simulink model "ARINC429_BNR"  (R2020b)
settings: Solver=VariableStepAuto  StartTime=0.0  StopTime=10.0  RelTol=1e-3
libraries: Bibavion x1
(part 2 of 3)

== system ARINC429_BNR/Decoder/De-serialize/Subsystem29 ==
  In1 : Inport
  Data Type Conversion5 : DataTypeConversion  OutDataTypeStr=uint32
  Data Type Conversion9 : DataTypeConversion  OutDataTypeStr=uint32
  Divide12 : Product  Inputs=*/
  Divide13 : Product  Inputs=*/  OutDataTypeStr=uint32
  Float Const : Constant  Value=2  OutDataTypeStr=single
  Float Const6 : Constant  Value=0.5  OutDataTypeStr=single
  Subtract5 : Sum  Inputs=+-
  Out1 : Outport
  Out2 : Outport  Port=2
  wires:
  Float Const/1 -> [F_2]
  Divide12/1 -> Subtract5/1, Data Type Conversion5/1
  Divide13/1 -> Data Type Conversion9/1
  Float Const6/1 -> Divide13/2
  Data Type Conversion5/1 -> Out2/1, Subtract5/2
  [F_2] -> Divide12/2
  Subtract5/1 -> Divide13/1
  Data Type Conversion9/1 -> Out1/1
  In1/1 -> Divide12/1

== system ARINC429_BNR/Decoder/De-serialize/Subsystem3 ==
  In1 : Inport
  Data Type Conversion5 : DataTypeConversion  OutDataTypeStr=uint32
  Data Type Conversion9 : DataTypeConversion  OutDataTypeStr=uint32
  Divide12 : Product  Inputs=*/  OutDataTypeStr=double
  Divide13 : Product  Inputs=*/
  Float Const : Constant  Value=2  OutDataTypeStr=single
  Float Const6 : Constant  Value=0.5  OutDataTypeStr=single
  Subtract5 : Sum  Inputs=+-
  Out1 : Outport
  Out2 : Outport  Port=2
  wires:
  Float Const/1 -> [F_2]
  Divide12/1 -> Subtract5/1, Data Type Conversion5/1
  Divide13/1 -> Data Type Conversion9/1
  Float Const6/1 -> Divide13/2
  Data Type Conversion5/1 -> Out2/1, Subtract5/2
  In1/1 -> Divide12/1
  [F_2] -> Divide12/2
  Subtract5/1 -> Divide13/1
  Data Type Conversion9/1 -> Out1/1

== system ARINC429_BNR/Decoder/De-serialize/Subsystem30 ==
  In1 : Inport
  Data Type Conversion5 : DataTypeConversion  OutDataTypeStr=uint32
  Data Type Conversion9 : DataTypeConversion  OutDataTypeStr=uint32
  Divide12 : Product  Inputs=*/
  Divide13 : Product  Inputs=*/  OutDataTypeStr=uint32
  Float Const : Constant  Value=2  OutDataTypeStr=single
  Float Const6 : Constant  Value=0.5  OutDataTypeStr=single
  Subtract5 : Sum  Inputs=+-
  Out1 : Outport
  Out2 : Outport  Port=2
  wires:
  Float Const/1 -> [F_2]
  Divide12/1 -> Subtract5/1, Data Type Conversion5/1
  Divide13/1 -> Data Type Conversion9/1
  Float Const6/1 -> Divide13/2
  Data Type Conversion5/1 -> Out2/1, Subtract5/2
  [F_2] -> Divide12/2
  Subtract5/1 -> Divide13/1
  Data Type Conversion9/1 -> Out1/1
  In1/1 -> Divide12/1

== system ARINC429_BNR/Decoder/De-serialize/Subsystem31 ==
  In1 : Inport
  Data Type Conversion5 : DataTypeConversion  OutDataTypeStr=uint32
  Data Type Conversion9 : DataTypeConversion  OutDataTypeStr=uint32
  Divide12 : Product  Inputs=*/
  Divide13 : Product  Inputs=*/  OutDataTypeStr=uint32
  Float Const : Constant  Value=2  OutDataTypeStr=single
  Float Const6 : Constant  Value=0.5  OutDataTypeStr=single
  Subtract5 : Sum  Inputs=+-
  Out1 : Outport
  Out2 : Outport  Port=2
  wires:
  Float Const/1 -> [F_2]
  Divide12/1 -> Subtract5/1, Data Type Conversion5/1
  Divide13/1 -> Data Type Conversion9/1
  Float Const6/1 -> Divide13/2
  Data Type Conversion5/1 -> Out2/1, Subtract5/2
  [F_2] -> Divide12/2
  Subtract5/1 -> Divide13/1
  Data Type Conversion9/1 -> Out1/1
  In1/1 -> Divide12/1

== system ARINC429_BNR/Decoder/De-serialize/Subsystem32 ==
  In1 : Inport
  Data Type Conversion5 : DataTypeConversion  OutDataTypeStr=uint32
  Data Type Conversion9 : DataTypeConversion  OutDataTypeStr=uint32
  Divide12 : Product  Inputs=*/
  Divide13 : Product  Inputs=*/  OutDataTypeStr=uint32
  Float Const : Constant  Value=2  OutDataTypeStr=single
  Float Const6 : Constant  Value=0.5  OutDataTypeStr=single
  Subtract5 : Sum  Inputs=+-
  Out1 : Outport
  Out2 : Outport  Port=2
  wires:
  Float Const/1 -> [F_2]
  Divide12/1 -> Subtract5/1, Data Type Conversion5/1
  Divide13/1 -> Data Type Conversion9/1
  Float Const6/1 -> Divide13/2
  Data Type Conversion5/1 -> Out2/1, Subtract5/2
  [F_2] -> Divide12/2
  Subtract5/1 -> Divide13/1
  Data Type Conversion9/1 -> Out1/1
  In1/1 -> Divide12/1

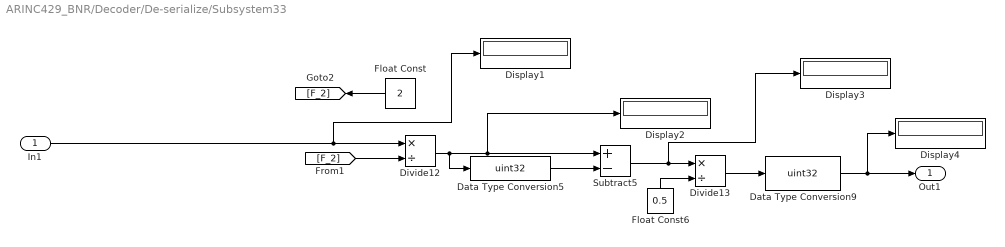
== system ARINC429_BNR/Decoder/De-serialize/Subsystem33 ==
  In1 : Inport
  Data Type Conversion5 : DataTypeConversion  OutDataTypeStr=uint32
  Data Type Conversion9 : DataTypeConversion  OutDataTypeStr=uint32
  Display{1..4} (4 alike) : Display
      settings: Format=decimal (Stored Integer)
  Divide12 : Product  Inputs=*/  OutDataTypeStr=double
  Divide13 : Product  Inputs=*/  OutDataTypeStr=uint32
  Float Const : Constant  Value=2  OutDataTypeStr=single
  Float Const6 : Constant  Value=0.5  OutDataTypeStr=single
  Subtract5 : Sum  Inputs=+-
  Out1 : Outport
  wires:
  Float Const/1 -> [F_2]
  Divide12/1 -> Display2/1, Subtract5/1, Data Type Conversion5/1
  Divide13/1 -> Data Type Conversion9/1
  Float Const6/1 -> Divide13/2
  Data Type Conversion5/1 -> Subtract5/2
  [F_2] -> Divide12/2
  Subtract5/1 -> Display3/1, Divide13/1
  Data Type Conversion9/1 -> Display4/1, Out1/1
  In1/1 -> Display1/1, Divide12/1

== system ARINC429_BNR/Decoder/De-serialize/Subsystem4 ==
  In1 : Inport
  Data Type Conversion5 : DataTypeConversion  OutDataTypeStr=uint32
  Data Type Conversion9 : DataTypeConversion  OutDataTypeStr=uint32
  Divide12 : Product  Inputs=*/  OutDataTypeStr=double
  Divide13 : Product  Inputs=*/  OutDataTypeStr=uint32
  Float Const : Constant  Value=2  OutDataTypeStr=single
  Float Const6 : Constant  Value=0.5  OutDataTypeStr=single
  Subtract5 : Sum  Inputs=+-
  Out1 : Outport
  Out2 : Outport  Port=2
  wires:
  Float Const/1 -> [F_2]
  Divide12/1 -> Subtract5/1, Data Type Conversion5/1
  Divide13/1 -> Data Type Conversion9/1
  Float Const6/1 -> Divide13/2
  Data Type Conversion5/1 -> Out2/1, Subtract5/2
  [F_2] -> Divide12/2
  Subtract5/1 -> Divide13/1
  Data Type Conversion9/1 -> Out1/1
  In1/1 -> Divide12/1

== system ARINC429_BNR/Decoder/De-serialize/Subsystem7 ==
  In1 : Inport
  Data Type Conversion5 : DataTypeConversion  OutDataTypeStr=uint32
  Data Type Conversion9 : DataTypeConversion  OutDataTypeStr=uint32
  Divide12 : Product  Inputs=*/  OutDataTypeStr=double
  Divide13 : Product  Inputs=*/  OutDataTypeStr=uint32
  Float Const : Constant  Value=2  OutDataTypeStr=single
  Float Const6 : Constant  Value=0.5  OutDataTypeStr=single
  Subtract5 : Sum  Inputs=+-
  Out1 : Outport
  Out2 : Outport  Port=2
  wires:
  Float Const/1 -> [F_2]
  Divide12/1 -> Subtract5/1, Data Type Conversion5/1
  Divide13/1 -> Data Type Conversion9/1
  Float Const6/1 -> Divide13/2
  Data Type Conversion5/1 -> Out2/1, Subtract5/2
  [F_2] -> Divide12/2
  Subtract5/1 -> Divide13/1
  Data Type Conversion9/1 -> Out1/1
  In1/1 -> Divide12/1

== system ARINC429_BNR/Decoder/De-serialize/Subsystem8 ==
  In1 : Inport
  Data Type Conversion5 : DataTypeConversion  OutDataTypeStr=uint32
  Data Type Conversion9 : DataTypeConversion  OutDataTypeStr=uint32
  Divide12 : Product  Inputs=*/  OutDataTypeStr=double
  Divide13 : Product  Inputs=*/  OutDataTypeStr=uint32
  Float Const : Constant  Value=2  OutDataTypeStr=single
  Float Const6 : Constant  Value=0.5  OutDataTypeStr=single
  Subtract5 : Sum  Inputs=+-
  Out1 : Outport
  Out2 : Outport  Port=2
  wires:
  Float Const/1 -> [F_2]
  Divide12/1 -> Subtract5/1, Data Type Conversion5/1
  Divide13/1 -> Data Type Conversion9/1
  Float Const6/1 -> Divide13/2
  Data Type Conversion5/1 -> Out2/1, Subtract5/2
  [F_2] -> Divide12/2
  Subtract5/1 -> Divide13/1
  Data Type Conversion9/1 -> Out1/1
  In1/1 -> Divide12/1

== system ARINC429_BNR/Decoder/De-serialize/Subsystem9 ==
  In1 : Inport
  Data Type Conversion5 : DataTypeConversion  OutDataTypeStr=uint32
  Data Type Conversion9 : DataTypeConversion  OutDataTypeStr=uint32
  Divide12 : Product  Inputs=*/  OutDataTypeStr=double
  Divide13 : Product  Inputs=*/  OutDataTypeStr=uint32
  Float Const : Constant  Value=2  OutDataTypeStr=single
  Float Const6 : Constant  Value=0.5  OutDataTypeStr=single
  Subtract5 : Sum  Inputs=+-
  Out1 : Outport
  Out2 : Outport  Port=2
  wires:
  Float Const/1 -> [F_2]
  Divide12/1 -> Subtract5/1, Data Type Conversion5/1
  Divide13/1 -> Data Type Conversion9/1
  Float Const6/1 -> Divide13/2
  Data Type Conversion5/1 -> Out2/1, Subtract5/2
  [F_2] -> Divide12/2
  Subtract5/1 -> Divide13/1
  Data Type Conversion9/1 -> Out1/1
  In1/1 -> Divide12/1

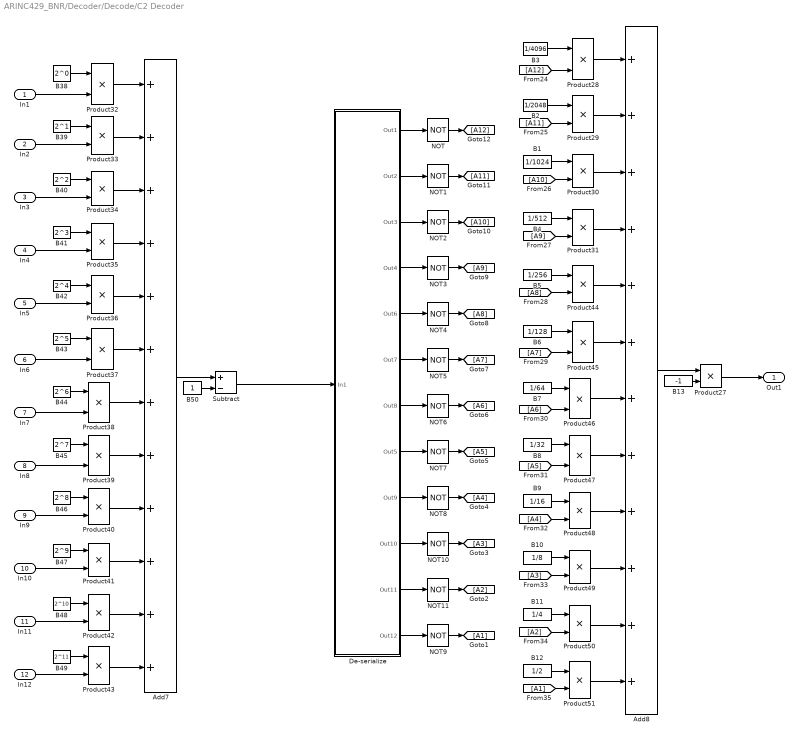
== system ARINC429_BNR/Decoder/Decode/C2 Decoder ==
  In1 : Inport
  In2 : Inport  Port=2
  In3 : Inport  Port=3
  In4 : Inport  Port=4
  In5 : Inport  Port=5
  In6 : Inport  Port=6
  In7 : Inport  Port=7
  In8 : Inport  Port=8
  In9 : Inport  Port=9
  In10 : Inport  Port=10
  In11 : Inport  Port=11
  In12 : Inport  Port=12
  Add7 : Sum  Inputs=++++++++++++  AccumDataTypeStr=uint32  OutDataTypeStr=uint32
  Add8 : Sum  Inputs=++++++++++++
  B1 : Constant  Value=1/1024  OutDataTypeStr=single
  B10 : Constant  Value=1/8  OutDataTypeStr=single
  B11 : Constant  Value=1/4  OutDataTypeStr=single
  B12 : Constant  Value=1/2  OutDataTypeStr=single
  B13 : Constant  Value=-1  OutDataTypeStr=single
  B2 : Constant  Value=1/2048  OutDataTypeStr=single
  B3 : Constant  Value=1/4096  OutDataTypeStr=single
  B38 : Constant  Value=2^0  OutDataTypeStr=single
  B39 : Constant  Value=2^1  OutDataTypeStr=single
  B4 : Constant  Value=1/512  OutDataTypeStr=single
  B40 : Constant  Value=2^2  OutDataTypeStr=single
  B41 : Constant  Value=2^3  OutDataTypeStr=single
  B42 : Constant  Value=2^4  OutDataTypeStr=single
  B43 : Constant  Value=2^5  OutDataTypeStr=single
  B44 : Constant  Value=2^6  OutDataTypeStr=single
  B45 : Constant  Value=2^7  OutDataTypeStr=single
  B46 : Constant  Value=2^8  OutDataTypeStr=single
  B47 : Constant  Value=2^9  OutDataTypeStr=single
  B48 : Constant  Value=2^10  OutDataTypeStr=single
  B49 : Constant  Value=2^11  OutDataTypeStr=single
  B5 : Constant  Value=1/256  OutDataTypeStr=single
  B50 : Constant  OutDataTypeStr=single
  B6 : Constant  Value=1/128  OutDataTypeStr=single
  B7 : Constant  Value=1/64  OutDataTypeStr=single
  B8 : Constant  Value=1/32  OutDataTypeStr=single
  B9 : Constant  Value=1/16  OutDataTypeStr=single
  De-serialize : Subsystem
  NOT{,1..11} (12 alike) : Logic  Operator=NOT  IconShape=distinctive  AllPortsSameDT=off  OutDataTypeStr=boolean
  Product{27..51} (25 alike) : Product
  Subtract : Sum  Inputs=+-
  Out1 : Outport
  wires:
  B41/1 -> Product35/1
  NOT1/1 -> [A11]
  De-serialize/12(Out12) -> NOT9/1
  [A12] -> Product28/2
  De-serialize/7(Out8) -> NOT6/1
  B48/1 -> Product42/1
  [A7] -> Product45/2
  Product30/1 -> Add8/3
  B44/1 -> Product38/1
  B42/1 -> Product36/1
  B49/1 -> Product43/1
  Product31/1 -> Add8/4
  Product42/1 -> Add7/11
  De-serialize/8(Out5) -> NOT7/1
  B46/1 -> Product40/1
  [A5] -> Product47/2
  NOT10/1 -> [A3]
  Product36/1 -> Add7/5
  B3/1 -> Product28/1
  NOT/1 -> [A12]
  Product41/1 -> Add7/10
  De-serialize/6(Out7) -> NOT5/1
  B45/1 -> Product39/1
  De-serialize/1(Out1) -> NOT/1
  NOT3/1 -> [A9]
  [A6] -> Product46/2
  Product44/1 -> Add8/5
  De-serialize/11(Out11) -> NOT11/1
  [A10] -> Product30/2
  Product35/1 -> Add7/4
  Product51/1 -> Add8/12
  Product43/1 -> Add7/12
  Product47/1 -> Add8/8
  In12/1 -> Product43/2
  NOT8/1 -> [A4]
  B11/1 -> Product50/1
  Subtract/1 -> De-serialize/1(In1)
  NOT2/1 -> [A10]
  [A1] -> Product51/2
  B38/1 -> Product32/1
  [A3] -> Product49/2
  B47/1 -> Product41/1
  De-serialize/4(Out4) -> NOT3/1
  Product37/1 -> Add7/6
  B1/1 -> Product30/1
  B9/1 -> Product48/1
  Product32/1 -> Add7/1
  Product34/1 -> Add7/3
  B39/1 -> Product33/1
  De-serialize/2(Out2) -> NOT1/1
  NOT9/1 -> [A1]
  De-serialize/3(Out3) -> NOT2/1
  [A9] -> Product31/2
  Product39/1 -> Add7/8
  Add7/1 -> Subtract/1
  [A11] -> Product29/2
  NOT11/1 -> [A2]
  B10/1 -> Product49/1
  B40/1 -> Product34/1
  B4/1 -> Product31/1
  Product33/1 -> Add7/2
  B50/1 -> Subtract/2
  NOT7/1 -> [A5]
  De-serialize/9(Out9) -> NOT8/1
  De-serialize/5(Out6) -> NOT4/1
  Product38/1 -> Add7/7
  B43/1 -> Product37/1
  Product40/1 -> Add7/9
  NOT5/1 -> [A7]
  B5/1 -> Product44/1
  B7/1 -> Product46/1
  Product48/1 -> Add8/9
  NOT4/1 -> [A8]
  De-serialize/10(Out10) -> NOT10/1
  B6/1 -> Product45/1
  Product46/1 -> Add8/7
  In2/1 -> Product33/2
  Product50/1 -> Add8/11
  Product45/1 -> Add8/6
  Product28/1 -> Add8/1
  Product29/1 -> Add8/2
  B8/1 -> Product47/1
  B12/1 -> Product51/1
  Product49/1 -> Add8/10
  [A2] -> Product50/2
  [A4] -> Product48/2
  B2/1 -> Product29/1
  [A8] -> Product44/2
  NOT6/1 -> [A6]
  In8/1 -> Product39/2
  In9/1 -> Product40/2
  In5/1 -> Product36/2
  In3/1 -> Product34/2
  In7/1 -> Product38/2
  In4/1 -> Product35/2
  In1/1 -> Product32/2
  In6/1 -> Product37/2
  In11/1 -> Product42/2
  In10/1 -> Product41/2
  Add8/1 -> Product27/1
  Product27/1 -> Out1/1
  B13/1 -> Product27/2

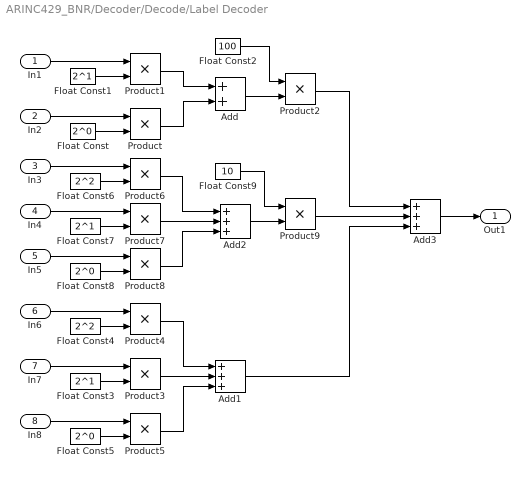
== system ARINC429_BNR/Decoder/Decode/Label Decoder ==
  In1 : Inport
  In2 : Inport  Port=2
  In3 : Inport  Port=3
  In4 : Inport  Port=4
  In5 : Inport  Port=5
  In6 : Inport  Port=6
  In7 : Inport  Port=7
  In8 : Inport  Port=8
  Add : Sum
  Add1 : Sum  Inputs=+++
  Add2 : Sum  Inputs=+++
  Add3 : Sum  Inputs=+++
  Float Const : Constant  Value=2^0  OutDataTypeStr=single
  Float Const1 : Constant  Value=2^1  OutDataTypeStr=single
  Float Const2 : Constant  Value=100  OutDataTypeStr=single
  Float Const3 : Constant  Value=2^1  OutDataTypeStr=single
  Float Const4 : Constant  Value=2^2  OutDataTypeStr=single
  Float Const5 : Constant  Value=2^0  OutDataTypeStr=single
  Float Const6 : Constant  Value=2^2  OutDataTypeStr=single
  Float Const7 : Constant  Value=2^1  OutDataTypeStr=single
  Float Const8 : Constant  Value=2^0  OutDataTypeStr=single
  Float Const9 : Constant  Value=10  OutDataTypeStr=single
  Product{,1..9} (10 alike) : Product
  Out1 : Outport
  wires:
  Product7/1 -> Add2/2
  In8/1 -> Product5/1
  Product3/1 -> Add1/2
  Float Const6/1 -> Product6/2
  In7/1 -> Product3/1
  Product/1 -> Add/2
  Float Const8/1 -> Product8/2
  In6/1 -> Product4/1
  Product9/1 -> Add3/2
  Add1/1 -> Add3/3
  Product4/1 -> Add1/1
  Float Const4/1 -> Product4/2
  Product6/1 -> Add2/1
  Float Const9/1 -> Product9/1
  Product8/1 -> Add2/3
  Float Const5/1 -> Product5/2
  Add2/1 -> Product9/2
  Float Const7/1 -> Product7/2
  Add/1 -> Product2/2
  Float Const/1 -> Product/2
  Product5/1 -> Add1/3
  In4/1 -> Product7/1
  Float Const2/1 -> Product2/1
  Float Const1/1 -> Product1/2
  Product1/1 -> Add/1
  Product2/1 -> Add3/1
  In1/1 -> Product1/1
  Float Const3/1 -> Product3/2
  In2/1 -> Product/1
  In5/1 -> Product8/1
  In3/1 -> Product6/1
  Add3/1 -> Out1/1

== system ARINC429_BNR/Decoder/Decode/SDI Decoder ==
  In1 : Inport
  In2 : Inport  Port=2
  Add4 : Sum
  Float Const10 : Constant  Value=2^0  OutDataTypeStr=single
  Float Const11 : Constant  Value=2^1  OutDataTypeStr=single
  Product10 : Product
  Product11 : Product
  Out1 : Outport
  wires:
  Product10/1 -> Add4/1
  Add4/1 -> Out1/1
  Product11/1 -> Add4/2
  Float Const11/1 -> Product11/2
  Float Const10/1 -> Product10/2
  In1/1 -> Product10/1
  In2/1 -> Product11/1

== system ARINC429_BNR/Decoder/Decode/SSM Decoder ==
  In1 : Inport
  In2 : Inport  Port=2
  Add5 : Sum
  Float Const12 : Constant  Value=2^0  OutDataTypeStr=single
  Float Const13 : Constant  Value=2^1  OutDataTypeStr=single
  Product12 : Product
  Product13 : Product
  Out1 : Outport
  wires:
  Product12/1 -> Add5/1
  Float Const13/1 -> Product13/2
  In2/1 -> Product13/1
  In1/1 -> Product12/1
  Product13/1 -> Add5/2
  Float Const12/1 -> Product12/2
  Add5/1 -> Out1/1

== system ARINC429_BNR/Encoder/Modulo10 /Subsystem ==
  In1 : Inport
  Data Type Conversion : DataTypeConversion  OutDataTypeStr=uint8
  Divide1 : Product  Inputs=*/
  Float Const2 : Constant  Value=10  OutDataTypeStr=single
  Product : Product
  Subtract : Sum  Inputs=+-
  Out1 : Outport
  Out2 : Outport  Port=2
  wires:
  Data Type Conversion/1 -> Out2/1, Subtract/2
  Float Const2/1 -> [F_10]
  Divide1/1 -> Subtract/1, Data Type Conversion/1
  Product/1 -> Out1/1
  Subtract/1 -> Product/1
  In1/1 -> Divide1/1
  [F_10] -> Divide1/2
  [F_10] -> Product/2

== system ARINC429_BNR/Encoder/Modulo10 /Subsystem1 ==
  In1 : Inport
  Data Type Conversion1 : DataTypeConversion  OutDataTypeStr=uint8
  Divide2 : Product  Inputs=*/
  Float Const2 : Constant  Value=10  OutDataTypeStr=single
  Product1 : Product
  Subtract1 : Sum  Inputs=+-
  Out1 : Outport
  Out2 : Outport  Port=2
  wires:
  Float Const2/1 -> [F_10]
  Data Type Conversion1/1 -> Out2/1, Subtract1/2
  In1/1 -> Divide2/1
  [F_10] -> Divide2/2
  [F_10] -> Product1/2
  Divide2/1 -> Subtract1/1, Data Type Conversion1/1
  Subtract1/1 -> Product1/1
  Product1/1 -> Out1/1

== system ARINC429_BNR/Encoder/Modulo10 /Subsystem2 ==
  In1 : Inport
  Data Type Conversion2 : DataTypeConversion  OutDataTypeStr=uint8
  Divide3 : Product  Inputs=*/
  Float Const1 : Constant  Value=10  OutDataTypeStr=single
  Product2 : Product
  Subtract2 : Sum  Inputs=+-
  Out1 : Outport
  wires:
  Product2/1 -> Out1/1
  [F_10] -> Product2/2
  In1/1 -> Divide3/1
  Data Type Conversion2/1 -> Subtract2/2
  Subtract2/1 -> Product2/1
  Divide3/1 -> Data Type Conversion2/1, Subtract2/1
  Float Const1/1 -> [F_10]
  [F_10] -> Divide3/2

== system ARINC429_BNR/Encoder/Subsystem12/Subsystem1 ==
  In1 : Inport
  In2 : Inport  Port=2
  Add8 : Sum  Inputs=-+
  B32 : Constant  Value=0  OutDataTypeStr=single
  Relational Operator4 : RelationalOperator  Operator=<=  OutDataTypeStr=boolean  RndMeth=Nearest
  Switch@0.3 : Switch  Threshold=0.5
  Out2 : Outport
  Out1 : Outport  Port=2
  wires:
  Add8/1 -> Switch@0.3/1, Relational Operator4/2
  Switch@0.3/1 -> Out2/1
  B32/1 -> Relational Operator4/1
  Relational Operator4/1 -> Out1/1, Switch@0.3/2
  In2/1 -> Add8/2, Switch@0.3/3
  In1/1 -> Add8/1

== system ARINC429_BNR/Encoder/Subsystem12/Subsystem10 ==
  In1 : Inport
  In2 : Inport  Port=2
  Add8 : Sum  Inputs=-+
  B32 : Constant  Value=0  OutDataTypeStr=single
  Relational Operator4 : RelationalOperator  Operator=<=  OutDataTypeStr=boolean  RndMeth=Nearest
  Switch@0.3 : Switch  Threshold=0.5
  Out2 : Outport
  Out1 : Outport  Port=2
  wires:
  Add8/1 -> Switch@0.3/1, Relational Operator4/2
  Switch@0.3/1 -> Out2/1
  B32/1 -> Relational Operator4/1
  Relational Operator4/1 -> Out1/1, Switch@0.3/2
  In2/1 -> Add8/2, Switch@0.3/3
  In1/1 -> Add8/1

== system ARINC429_BNR/Encoder/Subsystem12/Subsystem11 ==
  In1 : Inport
  In2 : Inport  Port=2
  Add8 : Sum  Inputs=-+
  B32 : Constant  Value=0  OutDataTypeStr=single
  Relational Operator4 : RelationalOperator  Operator=<=  OutDataTypeStr=boolean  RndMeth=Nearest
  Switch@0.3 : Switch  Threshold=0.5
  Out2 : Outport
  Out1 : Outport  Port=2
  wires:
  Add8/1 -> Switch@0.3/1, Relational Operator4/2
  Switch@0.3/1 -> Out2/1
  B32/1 -> Relational Operator4/1
  Relational Operator4/1 -> Out1/1, Switch@0.3/2
  In2/1 -> Add8/2, Switch@0.3/3
  In1/1 -> Add8/1

== system ARINC429_BNR/Encoder/Subsystem12/Subsystem12 ==
  In1 : Inport
  In2 : Inport  Port=2
  Add8 : Sum  Inputs=-+
  B32 : Constant  Value=0  OutDataTypeStr=single
  Relational Operator4 : RelationalOperator  Operator=<=  OutDataTypeStr=boolean  RndMeth=Nearest
  Switch@0.3 : Switch  Threshold=0.5
  Out2 : Outport
  Out1 : Outport  Port=2
  wires:
  Add8/1 -> Switch@0.3/1, Relational Operator4/2
  Switch@0.3/1 -> Out2/1
  B32/1 -> Relational Operator4/1
  Relational Operator4/1 -> Out1/1, Switch@0.3/2
  In2/1 -> Add8/2, Switch@0.3/3
  In1/1 -> Add8/1

== system ARINC429_BNR/Encoder/Subsystem12/Subsystem2 ==
  In1 : Inport
  In2 : Inport  Port=2
  Add8 : Sum  Inputs=-+
  B32 : Constant  Value=0  OutDataTypeStr=single
  Relational Operator4 : RelationalOperator  Operator=<=  OutDataTypeStr=boolean  RndMeth=Nearest
  Switch@0.3 : Switch  Threshold=0.5
  Out2 : Outport
  Out1 : Outport  Port=2
  wires:
  Add8/1 -> Switch@0.3/1, Relational Operator4/2
  Switch@0.3/1 -> Out2/1
  B32/1 -> Relational Operator4/1
  Relational Operator4/1 -> Out1/1, Switch@0.3/2
  In2/1 -> Add8/2, Switch@0.3/3
  In1/1 -> Add8/1

== system ARINC429_BNR/Encoder/Subsystem12/Subsystem3 ==
  In1 : Inport
  In2 : Inport  Port=2
  Add8 : Sum  Inputs=-+
  B32 : Constant  Value=0  OutDataTypeStr=single
  Relational Operator4 : RelationalOperator  Operator=<=  OutDataTypeStr=boolean  RndMeth=Nearest
  Switch@0.3 : Switch  Threshold=0.5
  Out2 : Outport
  Out1 : Outport  Port=2
  wires:
  Add8/1 -> Switch@0.3/1, Relational Operator4/2
  Switch@0.3/1 -> Out2/1
  B32/1 -> Relational Operator4/1
  Relational Operator4/1 -> Out1/1, Switch@0.3/2
  In2/1 -> Add8/2, Switch@0.3/3
  In1/1 -> Add8/1

== system ARINC429_BNR/Encoder/Subsystem12/Subsystem4 ==
  In1 : Inport
  In2 : Inport  Port=2
  Add8 : Sum  Inputs=-+
  B32 : Constant  Value=0  OutDataTypeStr=single
  Relational Operator4 : RelationalOperator  Operator=<=  OutDataTypeStr=boolean  RndMeth=Nearest
  Switch@0.3 : Switch  Threshold=0.5
  Out2 : Outport
  Out1 : Outport  Port=2
  wires:
  Add8/1 -> Switch@0.3/1, Relational Operator4/2
  Switch@0.3/1 -> Out2/1
  B32/1 -> Relational Operator4/1
  Relational Operator4/1 -> Out1/1, Switch@0.3/2
  In2/1 -> Add8/2, Switch@0.3/3
  In1/1 -> Add8/1

== system ARINC429_BNR/Encoder/Subsystem12/Subsystem5 ==
  In1 : Inport
  In2 : Inport  Port=2
  Add8 : Sum  Inputs=-+
  B32 : Constant  Value=0  OutDataTypeStr=single
  Relational Operator4 : RelationalOperator  Operator=<=  OutDataTypeStr=boolean  RndMeth=Nearest
  Switch@0.3 : Switch  Threshold=0.5
  Out2 : Outport
  Out1 : Outport  Port=2
  wires:
  Add8/1 -> Switch@0.3/1, Relational Operator4/2
  Switch@0.3/1 -> Out2/1
  B32/1 -> Relational Operator4/1
  Relational Operator4/1 -> Out1/1, Switch@0.3/2
  In2/1 -> Add8/2, Switch@0.3/3
  In1/1 -> Add8/1

== system ARINC429_BNR/Encoder/Subsystem12/Subsystem6 ==
  In1 : Inport
  In2 : Inport  Port=2
  Add8 : Sum  Inputs=-+
  B32 : Constant  Value=0  OutDataTypeStr=single
  Relational Operator4 : RelationalOperator  Operator=<=  OutDataTypeStr=boolean  RndMeth=Nearest
  Switch@0.3 : Switch  Threshold=0.5
  Out2 : Outport
  Out1 : Outport  Port=2
  wires:
  Add8/1 -> Switch@0.3/1, Relational Operator4/2
  Switch@0.3/1 -> Out2/1
  B32/1 -> Relational Operator4/1
  Relational Operator4/1 -> Out1/1, Switch@0.3/2
  In2/1 -> Add8/2, Switch@0.3/3
  In1/1 -> Add8/1

== system ARINC429_BNR/Encoder/Subsystem12/Subsystem7 ==
  In1 : Inport
  In2 : Inport  Port=2
  Add8 : Sum  Inputs=-+
  B32 : Constant  Value=0  OutDataTypeStr=single
  Relational Operator4 : RelationalOperator  Operator=<=  OutDataTypeStr=boolean  RndMeth=Nearest
  Switch@0.3 : Switch  Threshold=0.5
  Out2 : Outport
  Out1 : Outport  Port=2
  wires:
  Add8/1 -> Switch@0.3/1, Relational Operator4/2
  Switch@0.3/1 -> Out2/1
  B32/1 -> Relational Operator4/1
  Relational Operator4/1 -> Out1/1, Switch@0.3/2
  In2/1 -> Add8/2, Switch@0.3/3
  In1/1 -> Add8/1

== system ARINC429_BNR/Encoder/Subsystem12/Subsystem8 ==
  In1 : Inport
  In2 : Inport  Port=2
  Add8 : Sum  Inputs=-+
  B32 : Constant  Value=0  OutDataTypeStr=single
  Relational Operator4 : RelationalOperator  Operator=<=  OutDataTypeStr=boolean  RndMeth=Nearest
  Switch@0.3 : Switch  Threshold=0.5
  Out2 : Outport
  Out1 : Outport  Port=2
  wires:
  Add8/1 -> Switch@0.3/1, Relational Operator4/2
  Switch@0.3/1 -> Out2/1
  B32/1 -> Relational Operator4/1
  Relational Operator4/1 -> Out1/1, Switch@0.3/2
  In2/1 -> Add8/2, Switch@0.3/3
  In1/1 -> Add8/1

== system ARINC429_BNR/Encoder/Subsystem12/Subsystem9 ==
  In1 : Inport
  In2 : Inport  Port=2
  Add8 : Sum  Inputs=-+
  B32 : Constant  Value=0  OutDataTypeStr=single
  Relational Operator4 : RelationalOperator  Operator=<=  OutDataTypeStr=boolean  RndMeth=Nearest
  Switch@0.3 : Switch  Threshold=0.5
  Out2 : Outport
  Out1 : Outport  Port=2
  wires:
  Add8/1 -> Switch@0.3/1, Relational Operator4/2
  Switch@0.3/1 -> Out2/1
  B32/1 -> Relational Operator4/1
  Relational Operator4/1 -> Out1/1, Switch@0.3/2
  In2/1 -> Add8/2, Switch@0.3/3
  In1/1 -> Add8/1

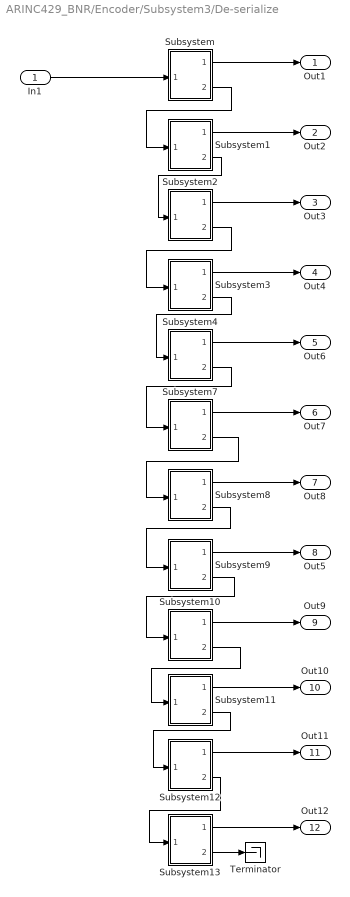
== system ARINC429_BNR/Encoder/Subsystem3/De-serialize ==
  In1 : Inport
  Subsystem : Subsystem
  Subsystem1 : Subsystem
  Subsystem10 : Subsystem
  Subsystem11 : Subsystem
  Subsystem12 : Subsystem
  Subsystem13 : Subsystem
  Subsystem2 : Subsystem
  Subsystem3 : Subsystem
  Subsystem4 : Subsystem
  Subsystem7 : Subsystem
  Subsystem8 : Subsystem
  Subsystem9 : Subsystem
  Terminator : Terminator
  Out1 : Outport
  Out2 : Outport  Port=2
  Out3 : Outport  Port=3
  Out4 : Outport  Port=4
  Out6 : Outport  Port=5
  Out7 : Outport  Port=6
  Out8 : Outport  Port=7
  Out5 : Outport  Port=8
  Out9 : Outport  Port=9
  Out10 : Outport  Port=10
  Out11 : Outport  Port=11
  Out12 : Outport  Port=12
  wires:
  Subsystem/1(Out1) -> Out1/1
  Subsystem1/1(Out1) -> Out2/1
  Subsystem1/2(Out2) -> Subsystem2/1(In1)
  Subsystem2/2(Out2) -> Subsystem3/1(In1)
  Subsystem3/2(Out2) -> Subsystem4/1(In1)
  Subsystem2/1(Out1) -> Out3/1
  Subsystem3/1(Out1) -> Out4/1
  Subsystem4/2(Out2) -> Subsystem7/1(In1)
  Subsystem4/1(Out1) -> Out6/1
  Subsystem7/1(Out1) -> Out7/1
  Subsystem8/1(Out1) -> Out8/1
  Subsystem10/2(Out2) -> Subsystem11/1(In1)
  Subsystem12/2(Out2) -> Subsystem13/1(In1)
  Subsystem11/2(Out2) -> Subsystem12/1(In1)
  Subsystem9/1(Out1) -> Out5/1
  Subsystem9/2(Out2) -> Subsystem10/1(In1)
  Subsystem10/1(Out1) -> Out9/1
  Subsystem11/1(Out1) -> Out10/1
  Subsystem12/1(Out1) -> Out11/1
  Subsystem13/1(Out1) -> Out12/1
  Subsystem7/2(Out2) -> Subsystem8/1(In1)
  Subsystem8/2(Out2) -> Subsystem9/1(In1)
  Subsystem/2(Out2) -> Subsystem1/1(In1)
  In1/1 -> Subsystem/1(In1)
  Subsystem13/2(Out2) -> Terminator/1

== system ARINC429_BNR/Encoder/base 8 encoder/Subsystem ==
  In1 : Inport
  Subsystem : Subsystem
  Subsystem1 : Subsystem
  Out1 : Outport
  Out2 : Outport  Port=2
  wires:
  In1/1 -> Subsystem/1(In1)
  Subsystem/1(Out1) -> Out1/1
  Subsystem/2(Out2) -> Subsystem1/1(In1)
  Subsystem1/1(Out1) -> Out2/1

== system ARINC429_BNR/Encoder/base 8 encoder/Subsystem1 ==
  In1 : Inport
  Subsystem : Subsystem
  Subsystem1 : Subsystem
  Subsystem2 : Subsystem
  Out1 : Outport
  Out2 : Outport  Port=2
  Out3 : Outport  Port=3
  wires:
  In1/1 -> Subsystem/1(In1)
  Subsystem/1(Out1) -> Out1/1
  Subsystem/2(Out2) -> Subsystem1/1(In1)
  Subsystem1/1(Out1) -> Out2/1
  Subsystem1/2(Out2) -> Subsystem2/1(In1)
  Subsystem2/1(Out1) -> Out3/1

== system ARINC429_BNR/Encoder/base 8 encoder/Subsystem2 ==
  In1 : Inport
  Subsystem : Subsystem
  Subsystem1 : Subsystem
  Subsystem2 : Subsystem
  Out1 : Outport
  Out2 : Outport  Port=2
  Out3 : Outport  Port=3
  wires:
  In1/1 -> Subsystem/1(In1)
  Subsystem/1(Out1) -> Out1/1
  Subsystem/2(Out2) -> Subsystem1/1(In1)
  Subsystem1/1(Out1) -> Out2/1
  Subsystem1/2(Out2) -> Subsystem2/1(In1)
  Subsystem2/1(Out1) -> Out3/1

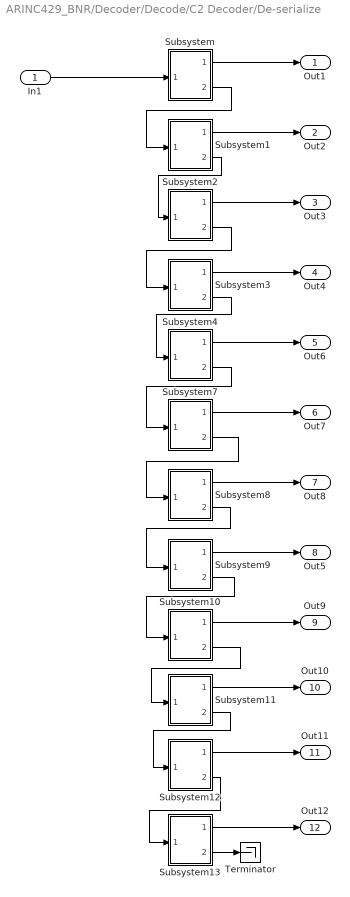
== system ARINC429_BNR/Decoder/Decode/C2 Decoder/De-serialize ==
  In1 : Inport
  Subsystem : Subsystem
  Subsystem1 : Subsystem
  Subsystem10 : Subsystem
  Subsystem11 : Subsystem
  Subsystem12 : Subsystem
  Subsystem13 : Subsystem
  Subsystem2 : Subsystem
  Subsystem3 : Subsystem
  Subsystem4 : Subsystem
  Subsystem7 : Subsystem
  Subsystem8 : Subsystem
  Subsystem9 : Subsystem
  Terminator : Terminator
  Out1 : Outport
  Out2 : Outport  Port=2
  Out3 : Outport  Port=3
  Out4 : Outport  Port=4
  Out6 : Outport  Port=5
  Out7 : Outport  Port=6
  Out8 : Outport  Port=7
  Out5 : Outport  Port=8
  Out9 : Outport  Port=9
  Out10 : Outport  Port=10
  Out11 : Outport  Port=11
  Out12 : Outport  Port=12
  wires:
  Subsystem/1(Out1) -> Out1/1
  Subsystem1/1(Out1) -> Out2/1
  Subsystem1/2(Out2) -> Subsystem2/1(In1)
  Subsystem2/2(Out2) -> Subsystem3/1(In1)
  Subsystem3/2(Out2) -> Subsystem4/1(In1)
  Subsystem2/1(Out1) -> Out3/1
  Subsystem3/1(Out1) -> Out4/1
  Subsystem4/2(Out2) -> Subsystem7/1(In1)
  Subsystem4/1(Out1) -> Out6/1
  Subsystem7/1(Out1) -> Out7/1
  Subsystem8/1(Out1) -> Out8/1
  Subsystem10/2(Out2) -> Subsystem11/1(In1)
  Subsystem12/2(Out2) -> Subsystem13/1(In1)
  Subsystem11/2(Out2) -> Subsystem12/1(In1)
  Subsystem9/1(Out1) -> Out5/1
  Subsystem9/2(Out2) -> Subsystem10/1(In1)
  Subsystem10/1(Out1) -> Out9/1
  Subsystem11/1(Out1) -> Out10/1
  Subsystem12/1(Out1) -> Out11/1
  Subsystem13/1(Out1) -> Out12/1
  Subsystem7/2(Out2) -> Subsystem8/1(In1)
  Subsystem8/2(Out2) -> Subsystem9/1(In1)
  Subsystem/2(Out2) -> Subsystem1/1(In1)
  In1/1 -> Subsystem/1(In1)
  Subsystem13/2(Out2) -> Terminator/1

== system ARINC429_BNR/Encoder/Subsystem3/De-serialize/Subsystem ==
  In1 : Inport
  Data Type Conversion5 : DataTypeConversion  OutDataTypeStr=uint32
  Data Type Conversion9 : DataTypeConversion  OutDataTypeStr=uint32
  Divide12 : Product  Inputs=*/  OutDataTypeStr=double
  Divide13 : Product  Inputs=*/  OutDataTypeStr=uint32
  Float Const : Constant  Value=2  OutDataTypeStr=single
  Float Const6 : Constant  Value=0.5  OutDataTypeStr=single
  Subtract5 : Sum  Inputs=+-
  Out1 : Outport
  Out2 : Outport  Port=2
  wires:
  Float Const/1 -> [F_2]
  Divide12/1 -> Subtract5/1, Data Type Conversion5/1
  Divide13/1 -> Data Type Conversion9/1
  Float Const6/1 -> Divide13/2
  Data Type Conversion5/1 -> Out2/1, Subtract5/2
  [F_2] -> Divide12/2
  Subtract5/1 -> Divide13/1
  Data Type Conversion9/1 -> Out1/1
  In1/1 -> Divide12/1

== system ARINC429_BNR/Encoder/Subsystem3/De-serialize/Subsystem1 ==
  In1 : Inport
  Data Type Conversion5 : DataTypeConversion  OutDataTypeStr=uint32
  Data Type Conversion9 : DataTypeConversion  OutDataTypeStr=uint32
  Divide12 : Product  Inputs=*/  OutDataTypeStr=double
  Divide13 : Product  Inputs=*/  OutDataTypeStr=uint32
  Float Const : Constant  Value=2  OutDataTypeStr=single
  Float Const6 : Constant  Value=0.5  OutDataTypeStr=single
  Subtract5 : Sum  Inputs=+-
  Out1 : Outport
  Out2 : Outport  Port=2
  wires:
  Float Const/1 -> [F_2]
  Divide12/1 -> Subtract5/1, Data Type Conversion5/1
  Divide13/1 -> Data Type Conversion9/1
  Float Const6/1 -> Divide13/2
  Data Type Conversion5/1 -> Out2/1, Subtract5/2
  [F_2] -> Divide12/2
  Subtract5/1 -> Divide13/1
  Data Type Conversion9/1 -> Out1/1
  In1/1 -> Divide12/1

== system ARINC429_BNR/Encoder/Subsystem3/De-serialize/Subsystem10 ==
  In1 : Inport
  Data Type Conversion5 : DataTypeConversion  OutDataTypeStr=uint32
  Data Type Conversion9 : DataTypeConversion  OutDataTypeStr=uint32
  Divide12 : Product  Inputs=*/  OutDataTypeStr=double
  Divide13 : Product  Inputs=*/  OutDataTypeStr=uint32
  Float Const : Constant  Value=2  OutDataTypeStr=single
  Float Const6 : Constant  Value=0.5  OutDataTypeStr=single
  Subtract5 : Sum  Inputs=+-
  Out1 : Outport
  Out2 : Outport  Port=2
  wires:
  Float Const/1 -> [F_2]
  Divide12/1 -> Subtract5/1, Data Type Conversion5/1
  Divide13/1 -> Data Type Conversion9/1
  Float Const6/1 -> Divide13/2
  Data Type Conversion5/1 -> Out2/1, Subtract5/2
  [F_2] -> Divide12/2
  Subtract5/1 -> Divide13/1
  Data Type Conversion9/1 -> Out1/1
  In1/1 -> Divide12/1

== system ARINC429_BNR/Encoder/Subsystem3/De-serialize/Subsystem11 ==
  In1 : Inport
  Data Type Conversion5 : DataTypeConversion  OutDataTypeStr=uint32
  Data Type Conversion9 : DataTypeConversion  OutDataTypeStr=uint32
  Divide12 : Product  Inputs=*/  OutDataTypeStr=double
  Divide13 : Product  Inputs=*/  OutDataTypeStr=uint32
  Float Const : Constant  Value=2  OutDataTypeStr=single
  Float Const6 : Constant  Value=0.5  OutDataTypeStr=single
  Subtract5 : Sum  Inputs=+-
  Out1 : Outport
  Out2 : Outport  Port=2
  wires:
  Float Const/1 -> [F_2]
  Divide12/1 -> Subtract5/1, Data Type Conversion5/1
  Divide13/1 -> Data Type Conversion9/1
  Float Const6/1 -> Divide13/2
  Data Type Conversion5/1 -> Out2/1, Subtract5/2
  [F_2] -> Divide12/2
  Subtract5/1 -> Divide13/1
  Data Type Conversion9/1 -> Out1/1
  In1/1 -> Divide12/1

== system ARINC429_BNR/Encoder/Subsystem3/De-serialize/Subsystem12 ==
  In1 : Inport
  Data Type Conversion5 : DataTypeConversion  OutDataTypeStr=uint32
  Data Type Conversion9 : DataTypeConversion  OutDataTypeStr=uint32
  Divide12 : Product  Inputs=*/  OutDataTypeStr=double
  Divide13 : Product  Inputs=*/  OutDataTypeStr=uint32
  Float Const : Constant  Value=2  OutDataTypeStr=single
  Float Const6 : Constant  Value=0.5  OutDataTypeStr=single
  Subtract5 : Sum  Inputs=+-
  Out1 : Outport
  Out2 : Outport  Port=2
  wires:
  Float Const/1 -> [F_2]
  Divide12/1 -> Subtract5/1, Data Type Conversion5/1
  Divide13/1 -> Data Type Conversion9/1
  Float Const6/1 -> Divide13/2
  Data Type Conversion5/1 -> Out2/1, Subtract5/2
  [F_2] -> Divide12/2
  Subtract5/1 -> Divide13/1
  Data Type Conversion9/1 -> Out1/1
  In1/1 -> Divide12/1

== system ARINC429_BNR/Encoder/Subsystem3/De-serialize/Subsystem13 ==
  In1 : Inport
  Data Type Conversion5 : DataTypeConversion  OutDataTypeStr=uint32
  Data Type Conversion9 : DataTypeConversion  OutDataTypeStr=uint32
  Divide12 : Product  Inputs=*/  OutDataTypeStr=double
  Divide13 : Product  Inputs=*/  OutDataTypeStr=uint32
  Float Const : Constant  Value=2  OutDataTypeStr=single
  Float Const6 : Constant  Value=0.5  OutDataTypeStr=single
  Subtract5 : Sum  Inputs=+-
  Out1 : Outport
  Out2 : Outport  Port=2
  wires:
  Float Const/1 -> [F_2]
  Divide12/1 -> Subtract5/1, Data Type Conversion5/1
  Divide13/1 -> Data Type Conversion9/1
  Float Const6/1 -> Divide13/2
  Data Type Conversion5/1 -> Out2/1, Subtract5/2
  [F_2] -> Divide12/2
  Subtract5/1 -> Divide13/1
  Data Type Conversion9/1 -> Out1/1
  In1/1 -> Divide12/1

== system ARINC429_BNR/Encoder/Subsystem3/De-serialize/Subsystem2 ==
  In1 : Inport
  Data Type Conversion5 : DataTypeConversion  OutDataTypeStr=uint32
  Data Type Conversion9 : DataTypeConversion  OutDataTypeStr=uint32
  Divide12 : Product  Inputs=*/  OutDataTypeStr=double
  Divide13 : Product  Inputs=*/  OutDataTypeStr=uint32
  Float Const : Constant  Value=2  OutDataTypeStr=single
  Float Const6 : Constant  Value=0.5  OutDataTypeStr=single
  Subtract5 : Sum  Inputs=+-
  Out1 : Outport
  Out2 : Outport  Port=2
  wires:
  Float Const/1 -> [F_2]
  Divide12/1 -> Subtract5/1, Data Type Conversion5/1
  Divide13/1 -> Data Type Conversion9/1
  Float Const6/1 -> Divide13/2
  Data Type Conversion5/1 -> Out2/1, Subtract5/2
  [F_2] -> Divide12/2
  Subtract5/1 -> Divide13/1
  Data Type Conversion9/1 -> Out1/1
  In1/1 -> Divide12/1

== system ARINC429_BNR/Encoder/Subsystem3/De-serialize/Subsystem3 ==
  In1 : Inport
  Data Type Conversion5 : DataTypeConversion  OutDataTypeStr=uint32
  Data Type Conversion9 : DataTypeConversion  OutDataTypeStr=uint32
  Divide12 : Product  Inputs=*/  OutDataTypeStr=double
  Divide13 : Product  Inputs=*/
  Float Const : Constant  Value=2  OutDataTypeStr=single
  Float Const6 : Constant  Value=0.5  OutDataTypeStr=single
  Subtract5 : Sum  Inputs=+-
  Out1 : Outport
  Out2 : Outport  Port=2
  wires:
  Float Const/1 -> [F_2]
  Divide12/1 -> Subtract5/1, Data Type Conversion5/1
  Divide13/1 -> Data Type Conversion9/1
  Float Const6/1 -> Divide13/2
  Data Type Conversion5/1 -> Out2/1, Subtract5/2
  In1/1 -> Divide12/1
  [F_2] -> Divide12/2
  Subtract5/1 -> Divide13/1
  Data Type Conversion9/1 -> Out1/1

== system ARINC429_BNR/Encoder/Subsystem3/De-serialize/Subsystem4 ==
  In1 : Inport
  Data Type Conversion5 : DataTypeConversion  OutDataTypeStr=uint32
  Data Type Conversion9 : DataTypeConversion  OutDataTypeStr=uint32
  Divide12 : Product  Inputs=*/  OutDataTypeStr=double
  Divide13 : Product  Inputs=*/  OutDataTypeStr=uint32
  Float Const : Constant  Value=2  OutDataTypeStr=single
  Float Const6 : Constant  Value=0.5  OutDataTypeStr=single
  Subtract5 : Sum  Inputs=+-
  Out1 : Outport
  Out2 : Outport  Port=2
  wires:
  Float Const/1 -> [F_2]
  Divide12/1 -> Subtract5/1, Data Type Conversion5/1
  Divide13/1 -> Data Type Conversion9/1
  Float Const6/1 -> Divide13/2
  Data Type Conversion5/1 -> Out2/1, Subtract5/2
  [F_2] -> Divide12/2
  Subtract5/1 -> Divide13/1
  Data Type Conversion9/1 -> Out1/1
  In1/1 -> Divide12/1

== system ARINC429_BNR/Encoder/Subsystem3/De-serialize/Subsystem7 ==
  In1 : Inport
  Data Type Conversion5 : DataTypeConversion  OutDataTypeStr=uint32
  Data Type Conversion9 : DataTypeConversion  OutDataTypeStr=uint32
  Divide12 : Product  Inputs=*/  OutDataTypeStr=double
  Divide13 : Product  Inputs=*/  OutDataTypeStr=uint32
  Float Const : Constant  Value=2  OutDataTypeStr=single
  Float Const6 : Constant  Value=0.5  OutDataTypeStr=single
  Subtract5 : Sum  Inputs=+-
  Out1 : Outport
  Out2 : Outport  Port=2
  wires:
  Float Const/1 -> [F_2]
  Divide12/1 -> Subtract5/1, Data Type Conversion5/1
  Divide13/1 -> Data Type Conversion9/1
  Float Const6/1 -> Divide13/2
  Data Type Conversion5/1 -> Out2/1, Subtract5/2
  [F_2] -> Divide12/2
  Subtract5/1 -> Divide13/1
  Data Type Conversion9/1 -> Out1/1
  In1/1 -> Divide12/1

== system ARINC429_BNR/Encoder/Subsystem3/De-serialize/Subsystem8 ==
  In1 : Inport
  Data Type Conversion5 : DataTypeConversion  OutDataTypeStr=uint32
  Data Type Conversion9 : DataTypeConversion  OutDataTypeStr=uint32
  Divide12 : Product  Inputs=*/  OutDataTypeStr=double
  Divide13 : Product  Inputs=*/  OutDataTypeStr=uint32
  Float Const : Constant  Value=2  OutDataTypeStr=single
  Float Const6 : Constant  Value=0.5  OutDataTypeStr=single
  Subtract5 : Sum  Inputs=+-
  Out1 : Outport
  Out2 : Outport  Port=2
  wires:
  Float Const/1 -> [F_2]
  Divide12/1 -> Subtract5/1, Data Type Conversion5/1
  Divide13/1 -> Data Type Conversion9/1
  Float Const6/1 -> Divide13/2
  Data Type Conversion5/1 -> Out2/1, Subtract5/2
  [F_2] -> Divide12/2
  Subtract5/1 -> Divide13/1
  Data Type Conversion9/1 -> Out1/1
  In1/1 -> Divide12/1

== system ARINC429_BNR/Encoder/Subsystem3/De-serialize/Subsystem9 ==
  In1 : Inport
  Data Type Conversion5 : DataTypeConversion  OutDataTypeStr=uint32
  Data Type Conversion9 : DataTypeConversion  OutDataTypeStr=uint32
  Divide12 : Product  Inputs=*/  OutDataTypeStr=double
  Divide13 : Product  Inputs=*/  OutDataTypeStr=uint32
  Float Const : Constant  Value=2  OutDataTypeStr=single
  Float Const6 : Constant  Value=0.5  OutDataTypeStr=single
  Subtract5 : Sum  Inputs=+-
  Out1 : Outport
  Out2 : Outport  Port=2
  wires:
  Float Const/1 -> [F_2]
  Divide12/1 -> Subtract5/1, Data Type Conversion5/1
  Divide13/1 -> Data Type Conversion9/1
  Float Const6/1 -> Divide13/2
  Data Type Conversion5/1 -> Out2/1, Subtract5/2
  [F_2] -> Divide12/2
  Subtract5/1 -> Divide13/1
  Data Type Conversion9/1 -> Out1/1
  In1/1 -> Divide12/1

== system ARINC429_BNR/Encoder/base 8 encoder/Subsystem/Subsystem ==
  In1 : Inport
  Data Type Conversion : DataTypeConversion  OutDataTypeStr=uint8
  Data Type Conversion15 : DataTypeConversion  OutDataTypeStr=uint8
  Divide1 : Product  Inputs=*/
  Divide2 : Product  Inputs=*/
  Float Const : Constant  Value=2  OutDataTypeStr=single
  Float Const1 : Constant  Value=0.5  OutDataTypeStr=single
  Subtract : Sum  Inputs=+-
  Out1 : Outport
  Out2 : Outport  Port=2
  wires:
  Data Type Conversion/1 -> Out2/1, Subtract/2
  Data Type Conversion15/1 -> Out1/1
  Float Const1/1 -> Divide2/2
  [F_2] -> Divide1/2
  Float Const/1 -> [F_2]
  Divide1/1 -> Subtract/1, Data Type Conversion/1
  In1/1 -> Divide1/1
  Subtract/1 -> Divide2/1
  Divide2/1 -> Data Type Conversion15/1

== system ARINC429_BNR/Encoder/base 8 encoder/Subsystem/Subsystem1 ==
  In1 : Inport
  Data Type Conversion1 : DataTypeConversion  OutDataTypeStr=uint8
  Data Type Conversion14 : DataTypeConversion  OutDataTypeStr=uint8
  Divide3 : Product  Inputs=*/
  Divide4 : Product  Inputs=*/
  Float Const : Constant  Value=1.99  OutDataTypeStr=single
  Float Const2 : Constant  Value=0.5  OutDataTypeStr=single
  Subtract2 : Sum  Inputs=+-
  Out1 : Outport
  wires:
  Divide3/1 -> Subtract2/1, Data Type Conversion1/1
  Data Type Conversion14/1 -> Out1/1
  [F_2] -> Divide3/2
  Divide4/1 -> Data Type Conversion14/1
  Subtract2/1 -> Divide4/1
  Float Const2/1 -> Divide4/2
  Data Type Conversion1/1 -> Subtract2/2
  In1/1 -> Divide3/1
  Float Const/1 -> [F_2]

== system ARINC429_BNR/Encoder/base 8 encoder/Subsystem1/Subsystem ==
  In1 : Inport
  Data Type Conversion2 : DataTypeConversion  OutDataTypeStr=uint8
  Data Type Conversion8 : DataTypeConversion  OutDataTypeStr=uint8
  Divide5 : Product  Inputs=*/
  Divide6 : Product  Inputs=*/
  Float Const : Constant  Value=1.99  OutDataTypeStr=single
  Float Const3 : Constant  Value=0.4999  OutDataTypeStr=single
  Subtract1 : Sum  Inputs=+-
  Out1 : Outport
  Out2 : Outport  Port=2
  wires:
  Divide5/1 -> Data Type Conversion2/1, Subtract1/1
  Float Const/1 -> [F_2]
  Divide6/1 -> Data Type Conversion8/1
  Data Type Conversion8/1 -> Out1/1
  Float Const3/1 -> Divide6/2
  Data Type Conversion2/1 -> Out2/1, Subtract1/2
  Subtract1/1 -> Divide6/1
  In1/1 -> Divide5/1
  [F_2] -> Divide5/2

== system ARINC429_BNR/Encoder/base 8 encoder/Subsystem1/Subsystem1 ==
  In1 : Inport
  Data Type Conversion13 : DataTypeConversion  OutDataTypeStr=uint8
  Data Type Conversion3 : DataTypeConversion  OutDataTypeStr=uint8
  Divide7 : Product  Inputs=*/
  Divide8 : Product  Inputs=*/
  Float Const : Constant  Value=1.99  OutDataTypeStr=single
  Float Const4 : Constant  Value=0.5  OutDataTypeStr=single
  Subtract3 : Sum  Inputs=+-
  Out1 : Outport
  Out2 : Outport  Port=2
  wires:
  Divide8/1 -> Data Type Conversion13/1
  Float Const4/1 -> Divide8/2
  Divide7/1 -> Subtract3/1, Data Type Conversion3/1
  [F_2] -> Divide7/2
  Subtract3/1 -> Divide8/1
  Data Type Conversion3/1 -> Out2/1, Subtract3/2
  In1/1 -> Divide7/1
  Data Type Conversion13/1 -> Out1/1
  Float Const/1 -> [F_2]

== system ARINC429_BNR/Encoder/base 8 encoder/Subsystem1/Subsystem2 ==
  In1 : Inport
  Data Type Conversion12 : DataTypeConversion  OutDataTypeStr=uint8
  Data Type Conversion4 : DataTypeConversion  OutDataTypeStr=uint8
  Divide10 : Product  Inputs=*/
  Divide9 : Product  Inputs=*/
  Float Const : Constant  Value=1.99  OutDataTypeStr=single
  Float Const5 : Constant  Value=0.5  OutDataTypeStr=single
  Subtract4 : Sum  Inputs=+-
  Out1 : Outport
  wires:
  In1/1 -> Divide9/1
  Subtract4/1 -> Divide10/1
  Divide9/1 -> Subtract4/1, Data Type Conversion4/1
  Divide10/1 -> Data Type Conversion12/1
  Float Const5/1 -> Divide10/2
  [F_2] -> Divide9/2
  Data Type Conversion12/1 -> Out1/1
  Float Const/1 -> [F_2]
  Data Type Conversion4/1 -> Subtract4/2

== system ARINC429_BNR/Encoder/base 8 encoder/Subsystem2/Subsystem ==
  In1 : Inport
  Data Type Conversion5 : DataTypeConversion  OutDataTypeStr=uint8
  Data Type Conversion9 : DataTypeConversion  OutDataTypeStr=uint8
  Divide12 : Product  Inputs=*/
  Divide13 : Product  Inputs=*/
  Float Const : Constant  Value=1.99  OutDataTypeStr=single
  Float Const6 : Constant  Value=0.50  OutDataTypeStr=single
  Subtract5 : Sum  Inputs=+-
  Out1 : Outport
  Out2 : Outport  Port=2
  wires:
  Divide12/1 -> Subtract5/1, Data Type Conversion5/1
  [F_2] -> Divide12/2
  Data Type Conversion9/1 -> Out1/1
  Data Type Conversion5/1 -> Out2/1, Subtract5/2
  Subtract5/1 -> Divide13/1
  Divide13/1 -> Data Type Conversion9/1
  In1/1 -> Divide12/1
  Float Const/1 -> [F_2]
  Float Const6/1 -> Divide13/2

== system ARINC429_BNR/Encoder/base 8 encoder/Subsystem2/Subsystem1 ==
  In1 : Inport
  Data Type Conversion10 : DataTypeConversion  OutDataTypeStr=uint8
  Data Type Conversion6 : DataTypeConversion  OutDataTypeStr=uint8
  Divide14 : Product  Inputs=*/
  Divide15 : Product  Inputs=*/
  Float Const : Constant  Value=1.99  OutDataTypeStr=single
  Float Const7 : Constant  Value=0.5  OutDataTypeStr=single
  Subtract6 : Sum  Inputs=+-
  Out1 : Outport
  Out2 : Outport  Port=2
  wires:
  Subtract6/1 -> Divide15/1
  Data Type Conversion6/1 -> Subtract6/2, Out2/1
  Float Const7/1 -> Divide15/2
  Divide14/1 -> Subtract6/1, Data Type Conversion6/1
  Divide15/1 -> Data Type Conversion10/1
  [F_2] -> Divide14/2
  In1/1 -> Divide14/1
  Data Type Conversion10/1 -> Out1/1
  Float Const/1 -> [F_2]

== system ARINC429_BNR/Encoder/base 8 encoder/Subsystem2/Subsystem2 ==
  In1 : Inport
  Data Type Conversion11 : DataTypeConversion  OutDataTypeStr=uint8
  Data Type Conversion7 : DataTypeConversion  OutDataTypeStr=uint8
  Divide11 : Product  Inputs=*/
  Divide16 : Product  Inputs=*/
  Float Const : Constant  Value=1.99  OutDataTypeStr=single
  Float Const8 : Constant  Value=0.49  OutDataTypeStr=single
  Subtract7 : Sum  Inputs=+-
  Out1 : Outport
  wires:
  Divide11/1 -> Data Type Conversion11/1
  Divide16/1 -> Subtract7/1, Data Type Conversion7/1
  Subtract7/1 -> Divide11/1
  [F_2] -> Divide16/2
  Float Const/1 -> [F_2]
  In1/1 -> Divide16/1
  Data Type Conversion7/1 -> Subtract7/2
  Float Const8/1 -> Divide11/2
  Data Type Conversion11/1 -> Out1/1

== system ARINC429_BNR/Decoder/Decode/C2 Decoder/De-serialize/Subsystem ==
  In1 : Inport
  Data Type Conversion5 : DataTypeConversion  OutDataTypeStr=uint32
  Data Type Conversion9 : DataTypeConversion  OutDataTypeStr=uint32
  Divide12 : Product  Inputs=*/  OutDataTypeStr=double
  Divide13 : Product  Inputs=*/  OutDataTypeStr=uint32
  Float Const : Constant  Value=2  OutDataTypeStr=single
  Float Const6 : Constant  Value=0.5  OutDataTypeStr=single
  Subtract5 : Sum  Inputs=+-
  Out1 : Outport
  Out2 : Outport  Port=2
  wires:
  Float Const/1 -> [F_2]
  Divide12/1 -> Subtract5/1, Data Type Conversion5/1
  Divide13/1 -> Data Type Conversion9/1
  Float Const6/1 -> Divide13/2
  Data Type Conversion5/1 -> Out2/1, Subtract5/2
  [F_2] -> Divide12/2
  Subtract5/1 -> Divide13/1
  Data Type Conversion9/1 -> Out1/1
  In1/1 -> Divide12/1

== system ARINC429_BNR/Decoder/Decode/C2 Decoder/De-serialize/Subsystem1 ==
  In1 : Inport
  Data Type Conversion5 : DataTypeConversion  OutDataTypeStr=uint32
  Data Type Conversion9 : DataTypeConversion  OutDataTypeStr=uint32
  Divide12 : Product  Inputs=*/  OutDataTypeStr=double
  Divide13 : Product  Inputs=*/  OutDataTypeStr=uint32
  Float Const : Constant  Value=2  OutDataTypeStr=single
  Float Const6 : Constant  Value=0.5  OutDataTypeStr=single
  Subtract5 : Sum  Inputs=+-
  Out1 : Outport
  Out2 : Outport  Port=2
  wires:
  Float Const/1 -> [F_2]
  Divide12/1 -> Subtract5/1, Data Type Conversion5/1
  Divide13/1 -> Data Type Conversion9/1
  Float Const6/1 -> Divide13/2
  Data Type Conversion5/1 -> Out2/1, Subtract5/2
  [F_2] -> Divide12/2
  Subtract5/1 -> Divide13/1
  Data Type Conversion9/1 -> Out1/1
  In1/1 -> Divide12/1

== system ARINC429_BNR/Decoder/Decode/C2 Decoder/De-serialize/Subsystem10 ==
  In1 : Inport
  Data Type Conversion5 : DataTypeConversion  OutDataTypeStr=uint32
  Data Type Conversion9 : DataTypeConversion  OutDataTypeStr=uint32
  Divide12 : Product  Inputs=*/  OutDataTypeStr=double
  Divide13 : Product  Inputs=*/  OutDataTypeStr=uint32
  Float Const : Constant  Value=2  OutDataTypeStr=single
  Float Const6 : Constant  Value=0.5  OutDataTypeStr=single
  Subtract5 : Sum  Inputs=+-
  Out1 : Outport
  Out2 : Outport  Port=2
  wires:
  Float Const/1 -> [F_2]
  Divide12/1 -> Subtract5/1, Data Type Conversion5/1
  Divide13/1 -> Data Type Conversion9/1
  Float Const6/1 -> Divide13/2
  Data Type Conversion5/1 -> Out2/1, Subtract5/2
  [F_2] -> Divide12/2
  Subtract5/1 -> Divide13/1
  Data Type Conversion9/1 -> Out1/1
  In1/1 -> Divide12/1

== system ARINC429_BNR/Decoder/Decode/C2 Decoder/De-serialize/Subsystem11 ==
  In1 : Inport
  Data Type Conversion5 : DataTypeConversion  OutDataTypeStr=uint32
  Data Type Conversion9 : DataTypeConversion  OutDataTypeStr=uint32
  Divide12 : Product  Inputs=*/  OutDataTypeStr=double
  Divide13 : Product  Inputs=*/  OutDataTypeStr=uint32
  Float Const : Constant  Value=2  OutDataTypeStr=single
  Float Const6 : Constant  Value=0.5  OutDataTypeStr=single
  Subtract5 : Sum  Inputs=+-
  Out1 : Outport
  Out2 : Outport  Port=2
  wires:
  Float Const/1 -> [F_2]
  Divide12/1 -> Subtract5/1, Data Type Conversion5/1
  Divide13/1 -> Data Type Conversion9/1
  Float Const6/1 -> Divide13/2
  Data Type Conversion5/1 -> Out2/1, Subtract5/2
  [F_2] -> Divide12/2
  Subtract5/1 -> Divide13/1
  Data Type Conversion9/1 -> Out1/1
  In1/1 -> Divide12/1

== system ARINC429_BNR/Decoder/Decode/C2 Decoder/De-serialize/Subsystem12 ==
  In1 : Inport
  Data Type Conversion5 : DataTypeConversion  OutDataTypeStr=uint32
  Data Type Conversion9 : DataTypeConversion  OutDataTypeStr=uint32
  Divide12 : Product  Inputs=*/  OutDataTypeStr=double
  Divide13 : Product  Inputs=*/  OutDataTypeStr=uint32
  Float Const : Constant  Value=2  OutDataTypeStr=single
  Float Const6 : Constant  Value=0.5  OutDataTypeStr=single
  Subtract5 : Sum  Inputs=+-
  Out1 : Outport
  Out2 : Outport  Port=2
  wires:
  Float Const/1 -> [F_2]
  Divide12/1 -> Subtract5/1, Data Type Conversion5/1
  Divide13/1 -> Data Type Conversion9/1
  Float Const6/1 -> Divide13/2
  Data Type Conversion5/1 -> Out2/1, Subtract5/2
  [F_2] -> Divide12/2
  Subtract5/1 -> Divide13/1
  Data Type Conversion9/1 -> Out1/1
  In1/1 -> Divide12/1

== system ARINC429_BNR/Decoder/Decode/C2 Decoder/De-serialize/Subsystem13 ==
  In1 : Inport
  Data Type Conversion5 : DataTypeConversion  OutDataTypeStr=uint32
  Data Type Conversion9 : DataTypeConversion  OutDataTypeStr=uint32
  Divide12 : Product  Inputs=*/  OutDataTypeStr=double
  Divide13 : Product  Inputs=*/  OutDataTypeStr=uint32
  Float Const : Constant  Value=2  OutDataTypeStr=single
  Float Const6 : Constant  Value=0.5  OutDataTypeStr=single
  Subtract5 : Sum  Inputs=+-
  Out1 : Outport
  Out2 : Outport  Port=2
  wires:
  Float Const/1 -> [F_2]
  Divide12/1 -> Subtract5/1, Data Type Conversion5/1
  Divide13/1 -> Data Type Conversion9/1
  Float Const6/1 -> Divide13/2
  Data Type Conversion5/1 -> Out2/1, Subtract5/2
  [F_2] -> Divide12/2
  Subtract5/1 -> Divide13/1
  Data Type Conversion9/1 -> Out1/1
  In1/1 -> Divide12/1
